simulink model "myTest"  (R2020a)
settings: Solver=FixedStepAuto  StartTime=0.0  StopTime=120  FixedStep=0.01  RelTol=1e-3
undefined symbols (not defined in the file or in its folder): serial
libraries: instrumentlib x2, aerolibanimutils x1, dspnetwork x1
settings Model: Creator=Admin  LastModifiedBy=Alireza
settings DataIOCC: ReturnWorkspaceOutputs=off
settings DebuggingCC: ArithmeticOperatorsInVariantConditions=warning
settings SFSimCC: SimUseLocalCustomCode=off  CustomCodeUndefinedFunction=UseInterfaceOnly
settings RTWCC: RTWUseLocalCustomCode=off
settings CodeAppCC: StateflowObjectComments=on

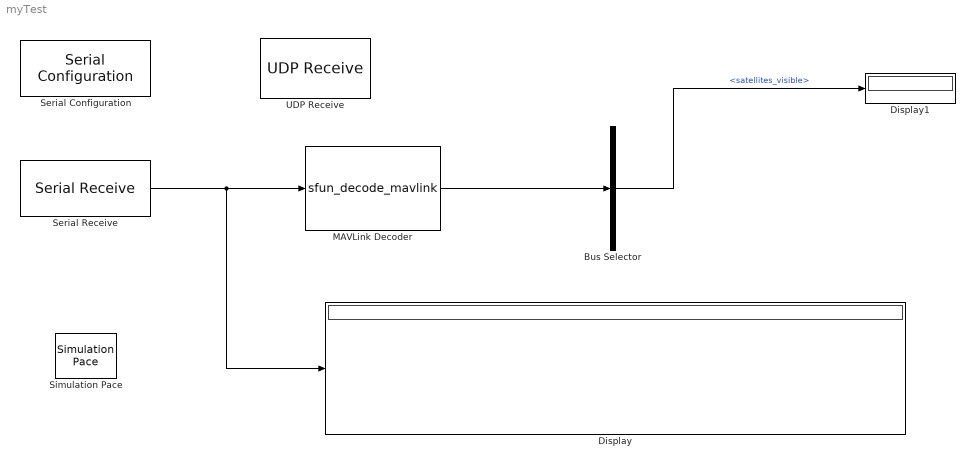
== system myTest ==
  Bus Selector : BusSelector  OutputSignals=satellites_visible
  Display : Display
  Display1 : Display
  MAVLink Decoder : S-Function  FunctionName=sfun_decode_mavlink  SFunctionDeploymentMode=off  EnableBusSupport=off
  Serial Configuration : instrumentlib/Serial Configuration  Priority=-200000  ComPortMenu=COM10  ComPort=COM10  ObjConstructor=serial('COM10');  BaudRate=115200  DataBits=8  Parity=none  StopBits=1  FlowControl=none  Timeout=10  ByteOrder=LittleEndian
  Serial Receive : instrumentlib/Serial Receive  ComPortMenu=COM10  ComPort=COM10  ObjConstructor=serial('COM10');  Terminator=<none>  DataSize=280  DataType=uint8  EnableBlockingMode=on  ActionDataUnavailable=Output last received value  CustomValue=0  SampleTime=0.01
  Simulation Pace : aerolibanimutils/Simulation Pace  SimulationPace=1  SleepMode=MATLAB Thread  OutputPaceError=off  SampleTime=0.01
  UDP Receive : dspnetwork/UDP Receive  localURL='0.0.0.0'  localPort=25000  remoteURL='0.0.0.0'  remotePort=-1  recvBufferSize=8192  dims=280  signalDatatype=uint8  isComplex=off  isVarSize=off  showBlockingTime=on  blockingTime=0  sampletime=0.01  blockPlatform=HOST
  wires:
  Serial Receive/1 -> Display/1, MAVLink Decoder/1
  MAVLink Decoder/1 -> Bus Selector/1
  Bus Selector/1 -> Display1/1  "<satellites_visible>"
